simulink model "MECOS_FW_sys"  (R2025b)
settings: Solver=VariableStepAuto  StartTime=0.0  StopTime=1.e-6  RelTol=1e-3
values from neighbouring files (symbols this model uses):
  FPGA_Ts = 1./FPGA_CLK    (= 8e-09)    [choPLL_loop_impl.m]
  FTW_nom_100kHz = round(Fref/FPGA_CLK*2^(Nbit_Cntr+1))    [choPLL_loop_impl.m]
  MECOS_A0 = 1./Bet0    [choPLL_loop_impl.m]
  MECOS_A1 = 2./Bet0    [choPLL_loop_impl.m]
  MECOS_A2 = 1./Bet0    [choPLL_loop_impl.m]
  MECOS_B1 = Bet1/Bet0    [choPLL_loop_impl.m]
  MECOS_B2 = Bet2/Bet0    [choPLL_loop_impl.m]
  MECOS_DF_gain = 0.25* (f_step*Nslits) / (FPGA_CLK/2^(Nbit_Cntr+1))    (= 0.369435906933)    [choPLL_loop_impl.m]
  Nbit_Cntr = 37    [choPLL_loop_impl.m]
libraries: hdlBasic x56, vmcUtilities x1, hdlUtilities x1
settings Model: Creator=valbas  LastModifiedBy=valbas
settings SolverCC: AlgebraicLoopSolver=TrustRegion
settings DebuggingCC: UnconnectedInputMsg=warning  UnconnectedOutputMsg=warning  UnconnectedLineMsg=warning
settings ModelReferenceCC: EnableRefExpFcnMdlSchedulingChecks=on
settings RTWCC: GPUComputeCapability=3.5  DLArmComputeVersion=19.05

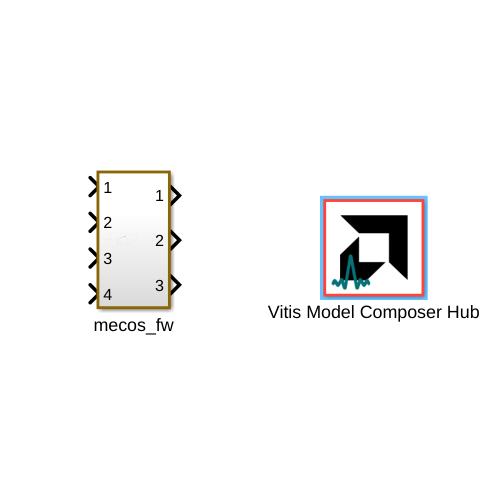
[thumbnail: Simulink's stored preview of the top-level diagram]
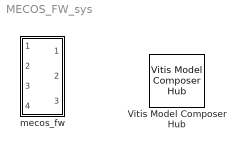
== system MECOS_FW_sys ==
  Vitis Model Composer Hub : vmcUtilities/Vitis Model Composer Hub  Tag=genX  CodeGeneration=off  SubsystemName=mecos_fw  BlockHierPath=MECOS_FW_sys/mecos_fw  CompilationType=HDLCompilation  SubsystemType=HDLNode  ExportTypeV2=IP Catalog  StartColumn=1  NumberOfColumns=1  TargetDirectory=./netlist  exportDesign=on  analyzeDesign=off  validateDesignOnHw=off  ExportType=HDL  IpVendor=xilinx.com  IpLibrary=hls  IpVersion=1.0  IpHWLanguage=Verilog  AieCompilerOptions={}  AieSimulatorOptions={}  CreateTestbench=off  TestbenchStackSize=10  RunRtlSim=off  RunCSim=off  RunAieSim=off  AieSimTimeout=50000  RunAieSimProfiling=off  LaunchVitisAnalyzer=off  PlotOutput=off  RunX86Sim=off  X86SimTimeout=10  GenHwImage=off  GenLibadfXo=on  GenHwValidationCode=off  PlatformType=Not Specified  HwSystemType=Baremetal  HwValidationTarget=hw  ProjDevice=Zynq UltraScale+ ZCU106 Evaluation Platform (xczu7ev-ffvc1156-2-e)  ProjDevicePart=xczu7ev-ffvc1156-2-e  AIEType=None  SamplePeriod=-1  ClockFrequency=200  DataPathParallelism=1  xilinxfamily=zynquplus  part=xczu7ev  speed=-2-e  package=ffvc1156  directory=./code/ip/mecos_fw/src  testbench=off  incr_netlist=off  synthesis_tool=Vivado  clock_wrapper=Clock Enables  dbl_ovrd=According to Block Masks  dcm_input_clock_period=10  sysclk_period=FPGA_Ts*1e9  simulink_period=FPGA_Ts  eval_field=0  IPInfoJsonString="{\"DUTSubsystemName\":\"mecos_fw\",\"HDLSubsystem\":{\"SubsystemName\":\"mecos_fw\",\"IPName\":\"mecos_fw\",\"IPLibrary\":\"ModelComp\",\"IPVendor\":\"MaxIV\",\"IPVersion\":\"1.2\",\"TargetDirectory\":\"./netlist\",\"SubsystemDir\":\"./netlist/ip/mecos_fw\",\"FreqHz\":\"125000000\"},\"SubsystemTag\":\"HDLNode\"}"  LogFileName=/xilinxworks/ZCU106/v2025.2/chopsync/gitcode/modelcomp/netlist/model_composer.log  NThreads=4  IPConfigFile=/tmp/vmctmp-5513881200898270237/MECOS_FW_sys_ipconfig.json
  mecos_fw : Subsystem

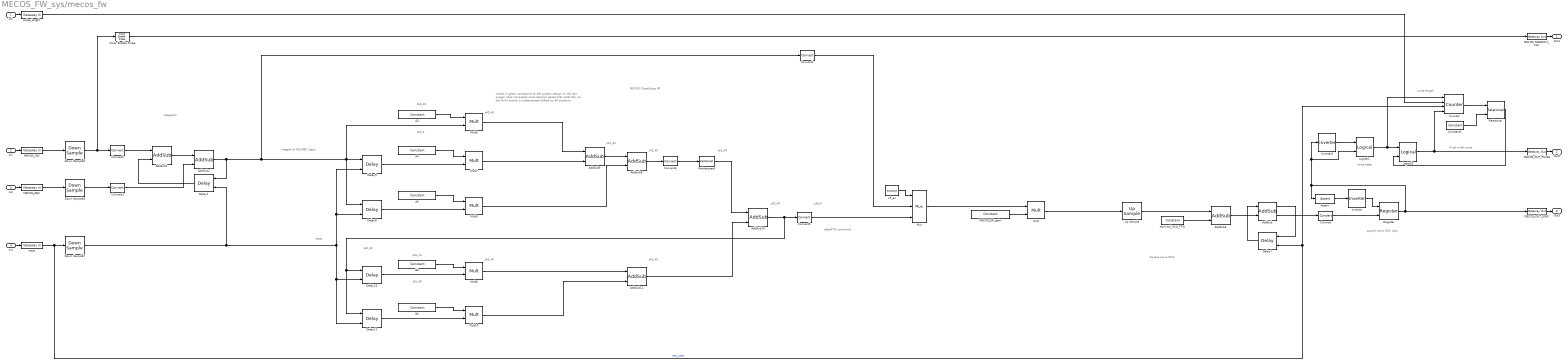
== system MECOS_FW_sys/mecos_fw ==
  note: pulse length
  note: Integrator
  note: Square-wave NCO
  note: s62_40
  note: s26_24
  note: s62_40
  note: s42_40
  note: s40_40
  note: s22_0
  note: s62_40
  note: s62_40
  note: integral of INC/DEC steps
  note: values in green correspond to the system design on the doc;
      | sysgen does not accept more decimal places than total bits,
      | so the AnXn branch is implemented shifted by 40 positions
  note: s18_40
  note: deltaFTW command
  note: MECOS ClosedLoop IIR
  note: s62_40
  note: s62_40
  note: s41_40
  note: reset
  note: s38_0
  note: rising edge
  note: fixed width pulse
  note: square wave 50% duty
  In1 : Inport
  In2 : Inport  Port=2
  In3 : Inport  Port=3
  In4 : Inport  Port=4
  A3 : hdlBasic/Constant  const=MECOS_A0*2^40  gui_display_data_type=Fixed-point  arith_type=Signed (2's comp)  n_bits=18  bin_pt=0  preci_type=Single  exp_width=8  frac_width=24  explicit_period=off  period=1  XmcBlockStatus=1  maskContainerNames=tabcontainer1  block_type=constant  block_config=sysgen:Constant_config
  A4 : hdlBasic/Constant  const=MECOS_A1*2^40  gui_display_data_type=Fixed-point  arith_type=Signed (2's comp)  n_bits=18  bin_pt=0  preci_type=Single  exp_width=8  frac_width=24  explicit_period=off  period=1  XmcBlockStatus=1  maskContainerNames=tabcontainer1  block_type=constant  block_config=sysgen:Constant_config
  A5 : hdlBasic/Constant  const=MECOS_A2*2^40  gui_display_data_type=Fixed-point  arith_type=Signed (2's comp)  n_bits=18  bin_pt=0  preci_type=Single  exp_width=8  frac_width=24  explicit_period=off  period=1  XmcBlockStatus=1  maskContainerNames=tabcontainer1  block_type=constant  block_config=sysgen:Constant_config
  AddSub : hdlBasic/AddSub  mode=Addition  use_carryin=off  use_carryout=on  en=off  latency=0  precision=User Defined  arith_type=Unsigned  n_bits=Nbit_Cntr  bin_pt=0  quantization=Truncate  overflow=Wrap  use_behavioral_HDL=off  hw_selection=Fabric  pipelined=off  XmcBlockStatus=1  maskContainerNames=tabcontainer1  block_type=addsub  block_config=sysgen:Addsub_config
  AddSub1 : hdlBasic/AddSub  mode=Addition  use_carryin=off  use_carryout=off  en=off  latency=0  precision=User Defined  arith_type="Signed  (2's comp)"  n_bits=22  bin_pt=0  quantization="Round  (unbiased: +/- Inf)"  overflow=Saturate  use_behavioral_HDL=off  hw_selection=Fabric  pipelined=off  XmcBlockStatus=1  maskContainerNames=tabcontainer1  block_type=addsub  block_config=sysgen:Addsub_config
  AddSub10 : hdlBasic/AddSub  mode=Subtraction  use_carryin=off  use_carryout=off  en=off  latency=0  precision=User Defined  arith_type="Signed  (2's comp)"  n_bits=62  bin_pt=40  quantization="Round  (unbiased: +/- Inf)"  overflow=Saturate  use_behavioral_HDL=off  hw_selection=Fabric  pipelined=off  XmcBlockStatus=1  maskContainerNames=tabcontainer1  block_type=addsub  block_config=sysgen:Addsub_config
  AddSub11 : hdlBasic/AddSub  mode=Addition  use_carryin=off  use_carryout=off  en=off  latency=0  precision=User Defined  arith_type="Signed  (2's comp)"  n_bits=62  bin_pt=40  quantization="Round  (unbiased: +/- Inf)"  overflow=Saturate  use_behavioral_HDL=off  hw_selection=Fabric  pipelined=off  XmcBlockStatus=1  maskContainerNames=tabcontainer1  block_type=addsub  block_config=sysgen:Addsub_config
  AddSub2 : hdlBasic/AddSub  mode=Subtraction  use_carryin=off  use_carryout=off  en=off  latency=0  precision=User Defined  arith_type="Signed  (2's comp)"  n_bits=22  bin_pt=0  quantization="Round  (unbiased: +/- Inf)"  overflow=Saturate  use_behavioral_HDL=off  hw_selection=Fabric  pipelined=off  XmcBlockStatus=1  maskContainerNames=tabcontainer1  block_type=addsub  block_config=sysgen:Addsub_config
  AddSub3 : hdlBasic/AddSub  mode=Addition  use_carryin=off  use_carryout=off  en=off  latency=1  precision=User Defined  arith_type=Unsigned  n_bits=Nbit_Cntr  bin_pt=0  quantization=Truncate  overflow=Saturate  use_behavioral_HDL=off  hw_selection=Fabric  pipelined=off  XmcBlockStatus=1  maskContainerNames=tabcontainer1  block_type=addsub  block_config=sysgen:Addsub_config
  AddSub8 : hdlBasic/AddSub  mode=Addition  use_carryin=off  use_carryout=off  en=off  latency=0  precision=Full  arith_type=Unsigned  n_bits=16  bin_pt=14  quantization=Truncate  overflow=Wrap  use_behavioral_HDL=off  hw_selection=Fabric  pipelined=off  XmcBlockStatus=1  maskContainerNames=tabcontainer1  block_type=addsub  block_config=sysgen:Addsub_config
  AddSub9 : hdlBasic/AddSub  mode=Addition  use_carryin=off  use_carryout=off  en=off  latency=0  precision=Full  arith_type=Unsigned  n_bits=16  bin_pt=14  quantization=Truncate  overflow=Wrap  use_behavioral_HDL=off  hw_selection=Fabric  pipelined=off  XmcBlockStatus=1  maskContainerNames=tabcontainer1  block_type=addsub  block_config=sysgen:Addsub_config
  Assert : hdlBasic/Assert  assert_type=on  type_source=Explicitly  gui_display_data_type=Boolean  arith_type=Boolean  n_bits=16  bin_pt=14  preci_type=Single  exp_width=8  frac_width=24  assert_rate=off  rate_source=Explicitly  period=1  output_port=on  XmcBlockStatus=1  maskContainerNames=group1  block_type=assert  block_config=sysgen:assert_config  block_width=609  block_height=900
  B3 : hdlBasic/Constant  const=MECOS_B1  gui_display_data_type=Fixed-point  arith_type=Signed (2's comp)  n_bits=26  bin_pt=24  preci_type=Single  exp_width=8  frac_width=24  explicit_period=off  period=1  XmcBlockStatus=1  maskContainerNames=tabcontainer1  block_type=constant  block_config=sysgen:Constant_config
  B4 : hdlBasic/Constant  const=MECOS_B2  gui_display_data_type=Fixed-point  arith_type=Signed (2's comp)  n_bits=26  bin_pt=24  preci_type=Single  exp_width=8  frac_width=24  explicit_period=off  period=1  XmcBlockStatus=1  maskContainerNames=tabcontainer1  block_type=constant  block_config=sysgen:Constant_config
  Clock Enable Probe : hdlUtilities/Clock Enable Probe  inherit_constraints=on  XmcBlockStatus=1  maskContainerNames=group1  block_type=ceprobe  block_config=sysgen:CEProbe_config
  Constant1 : hdlBasic/Constant  const=0  gui_display_data_type=Fixed-point  arith_type=Unsigned  n_bits=10  bin_pt=0  preci_type=Single  exp_width=8  frac_width=24  explicit_period=off  period=1  XmcBlockStatus=1  maskContainerNames=tabcontainer1  block_type=constant  block_config=sysgen:Constant_config
  Convert : hdlBasic/Convert  gui_display_data_type=Boolean  arith_type=Boolean  n_bits=16  bin_pt=14  float_type=Single  exp_bits=8  fraction_bits=24  quantization=Truncate  overflow=Wrap  en=off  latency=1  pipeline=off  XmcBlockStatus=1  maskContainerNames=group2  block_type=convert  block_config=sysgen:Convert_config  block_width=595  block_height=885
  Convert1 : hdlBasic/Convert  gui_display_data_type=Fixed-point  arith_type=Signed (2's comp)  n_bits=38  bin_pt=0  float_type=Single  exp_bits=8  fraction_bits=24  quantization="Round  (unbiased: Even Values)"  overflow=Saturate  en=off  latency=1  pipeline=off  XmcBlockStatus=1  maskContainerNames=group2  block_type=convert  block_config=sysgen:Convert_config  block_width=595  block_height=885
  Convert2 : hdlBasic/Convert  gui_display_data_type=Fixed-point  arith_type=Signed (2's comp)  n_bits=22  bin_pt=0  float_type=Single  exp_bits=8  fraction_bits=24  quantization=Truncate  overflow=Wrap  en=off  latency=0  pipeline=off  XmcBlockStatus=1  maskContainerNames=group2  block_type=convert  block_config=sysgen:Convert_config  block_width=595  block_height=885
  Convert3 : hdlBasic/Convert  gui_display_data_type=Fixed-point  arith_type=Signed (2's comp)  n_bits=22  bin_pt=0  float_type=Single  exp_bits=8  fraction_bits=24  quantization=Truncate  overflow=Wrap  en=off  latency=0  pipeline=off  XmcBlockStatus=1  maskContainerNames=group2  block_type=convert  block_config=sysgen:Convert_config  block_width=595  block_height=885
  Convert5 : hdlBasic/Convert  gui_display_data_type=Fixed-point  arith_type=Signed (2's comp)  n_bits=38  bin_pt=0  float_type=Single  exp_bits=8  fraction_bits=24  quantization="Round  (unbiased: Even Values)"  overflow=Saturate  en=off  latency=1  pipeline=off  XmcBlockStatus=1  maskContainerNames=group2  block_type=convert  block_config=sysgen:Convert_config  block_width=595  block_height=885
  Convert6 : hdlBasic/Convert  gui_display_data_type=Fixed-point  arith_type=Signed (2's comp)  n_bits=62  bin_pt=0  float_type=Single  exp_bits=8  fraction_bits=24  quantization="Round  (unbiased: Even Values)"  overflow=Saturate  en=off  latency=0  pipeline=off  XmcBlockStatus=1  maskContainerNames=group2  block_type=convert  block_config=sysgen:Convert_config  block_width=595  block_height=885
  Counter : hdlBasic/Counter  cnt_type=Free running  cnt_to=Inf  operation=Down  start_count=1  cnt_by_val=1  arith_type=Unsigned  n_bits=10  bin_pt=0  load_pin=on  rst=on  en=on  explicit_period=Explicit  period=FPGA_Ts  use_behavioral_HDL=off  implementation=Fabric  XmcBlockStatus=1  maskContainerNames=group1  block_type=counter  block_config=sysgen:Counter_config  block_width=531  block_height=1023
  Delay{2,7,9..10} (4 alike) : hdlBasic/Delay  rst=on  en=off  latency=1  reg_retiming=off  XmcBlockStatus=1  maskContainerNames=group1  block_type=delay  block_config=sysgen:Delay_config
  Delay11 : hdlBasic/Delay  rst=on  en=off  latency=2  reg_retiming=off  XmcBlockStatus=1  maskContainerNames=group1  block_type=delay  block_config=sysgen:Delay_config
  Delay8 : hdlBasic/Delay  rst=on  en=off  latency=2  reg_retiming=off  XmcBlockStatus=1  maskContainerNames=group1  block_type=delay  block_config=sysgen:Delay_config
  Down Sample5 : hdlBasic/Down Sample  sample_ratio=MECOS_dec  sample_phase="Last Value of Frame  (most efficient)"  en=off  rst=off  latency=1  XmcBlockStatus=1  maskContainerNames=group1  block_type=dsamp  block_config=sysgen:Downsample_config
  Down Sample6 : hdlBasic/Down Sample  sample_ratio=MECOS_dec  sample_phase="Last Value of Frame  (most efficient)"  en=off  rst=off  latency=1  XmcBlockStatus=1  maskContainerNames=group1  block_type=dsamp  block_config=sysgen:Downsample_config
  Down Sample7 : hdlBasic/Down Sample  sample_ratio=MECOS_dec  sample_phase="Last Value of Frame  (most efficient)"  en=off  rst=off  latency=1  XmcBlockStatus=1  maskContainerNames=group1  block_type=dsamp  block_config=sysgen:Downsample_config
  Inverter : hdlBasic/Inverter  en=off  latency=1  XmcBlockStatus=1  maskContainerNames=group2  block_type=inv  block_config=sysgen:Inverter_config
  Inverter3 : hdlBasic/Inverter  en=off  latency=1  XmcBlockStatus=1  maskContainerNames=group2  block_type=inv  block_config=sysgen:Inverter_config
  LP_en : hdlBasic/Constant  const=1  gui_display_data_type=Boolean  arith_type=Boolean  n_bits=18  bin_pt=0  preci_type=Single  exp_width=8  frac_width=24  explicit_period=off  period=1  XmcBlockStatus=1  maskContainerNames=tabcontainer1  block_type=constant  block_config=sysgen:Constant_config
  Logical1 : hdlBasic/Logical  logical_function=AND  inputs=2  en=off  latency=0  precision=Full  arith_type=Unsigned  n_bits=16  bin_pt=0  align_bp=on  overflow=[]  quantization=[]  XmcBlockStatus=1  maskContainerNames=tabcontainer1  block_type=logical  block_config=sysgen:Logical_config
  Logical3 : hdlBasic/Logical  logical_function=OR  inputs=2  en=off  latency=0  precision=Full  arith_type=Unsigned  n_bits=16  bin_pt=0  align_bp=on  overflow=[]  quantization=[]  XmcBlockStatus=1  maskContainerNames=tabcontainer1  block_type=logical  block_config=sysgen:Logical_config
  MECOS_DEC : hdlBasic/Gateway In  gui_display_data_type=Boolean  arith_type=Boolean  n_bits=16  bin_pt=14  preci_type=Single  exp_width=8  frac_width=24  rows=1  columns=1  quantization="Round  (unbiased: +/- Inf)"  overflow=Saturate  period=FPGA_Ts  UseAsADC=off  ADCChannel='1'  interface=None  automatic_assignment=on  address_offset=hex2dec('00')  intf_name=''  intf_description=''  default_value=0  timing_constraint=None  locs_specified=off  LOCs={}  io_standard={}  inherit_from_input=off  hdl_port=on  XmcBlockStatus=1  maskContainerNames=group4  block_type=gatewayin  block_config=sysgen:gateway_in_config  block_width_w=590  block_height_w=620  block_width=640  block_height=850
  MECOS_DF_gain : hdlBasic/Constant  const=MECOS_DF_gain  gui_display_data_type=Fixed-point  arith_type=Signed (2's comp)  n_bits=18  bin_pt=15  preci_type=Single  exp_width=8  frac_width=24  explicit_period=off  period=1  XmcBlockStatus=1  maskContainerNames=tabcontainer1  block_type=constant  block_config=sysgen:Constant_config
  MECOS_INC : hdlBasic/Gateway In  gui_display_data_type=Boolean  arith_type=Boolean  n_bits=16  bin_pt=14  preci_type=Single  exp_width=8  frac_width=24  rows=1  columns=1  quantization="Round  (unbiased: +/- Inf)"  overflow=Saturate  period=FPGA_Ts  UseAsADC=off  ADCChannel='1'  interface=None  automatic_assignment=on  address_offset=hex2dec('00')  intf_name=''  intf_description=''  default_value=0  timing_constraint=None  locs_specified=off  LOCs={}  io_standard={}  inherit_from_input=off  hdl_port=on  XmcBlockStatus=1  maskContainerNames=group4  block_type=gatewayin  block_config=sysgen:gateway_in_config  block_width_w=590  block_height_w=620  block_width=640  block_height=850
  MECOS_OUT_PULSE : hdlBasic/Gateway Out  inherit_from_input=off  bool_to_boolean=off  hdl_port=on  rows=1  columns=1  UseAsDAC=off  DACChannel='1'  interface=None  automatic_assignment=on  address_offset=hex2dec('00')  intf_name=''  intf_description=''  timing_constraint=None  locs_specified=off  LOCs={}  io_standard={}  XmcBlockStatus=1  maskContainerNames=group4  block_type=gatewayout  block_config=sysgen:gateway_out_config  block_width_w=590  block_height_w=620  block_width=620  block_height=750
  MECOS_OUT_SQW : hdlBasic/Gateway Out  inherit_from_input=off  bool_to_boolean=off  hdl_port=on  rows=1  columns=1  UseAsDAC=off  DACChannel='1'  interface=None  automatic_assignment=on  address_offset=hex2dec('00')  intf_name=''  intf_description=''  timing_constraint=None  locs_specified=off  LOCs={}  io_standard={}  XmcBlockStatus=1  maskContainerNames=group4  block_type=gatewayout  block_config=sysgen:gateway_out_config  block_width_w=590  block_height_w=620  block_width=620  block_height=750
  MECOS_READOUT_CLK : hdlBasic/Gateway Out  inherit_from_input=off  bool_to_boolean=off  hdl_port=on  rows=1  columns=1  UseAsDAC=off  DACChannel='1'  interface=None  automatic_assignment=on  address_offset=hex2dec('00')  intf_name=''  intf_description=''  timing_constraint=None  locs_specified=off  LOCs={}  io_standard={}  XmcBlockStatus=1  maskContainerNames=group4  block_type=gatewayout  block_config=sysgen:gateway_out_config  block_width_w=590  block_height_w=620  block_width=620  block_height=750
  Mult : hdlBasic/Mult  precision=User Defined  arith_type="Signed  (2's comp)"  n_bits=38  bin_pt=0  quantization="Round  (unbiased: +/- Inf)"  overflow=Saturate  en=off  latency=0  opt_float=off  fp_mult_usage=No Usage  use_behavioral_HDL=off  opt=Speed  use_embedded=on  optimum_pipeline=off  pipeline=on  use_rpm=on  placement_style=Triangular  XmcBlockStatus=1  maskContainerNames=group1  block_type=mult  block_config=sysgen:Mult_config  block_width=598  block_height=876
  Mult10 : hdlBasic/Mult  precision=User Defined  arith_type="Signed  (2's comp)"  n_bits=62  bin_pt=40  quantization="Round  (unbiased: +/- Inf)"  overflow=Saturate  en=off  latency=0  opt_float=off  fp_mult_usage=No Usage  use_behavioral_HDL=off  opt=Speed  use_embedded=on  optimum_pipeline=off  pipeline=on  use_rpm=on  placement_style=Triangular  XmcBlockStatus=1  maskContainerNames=group1  block_type=mult  block_config=sysgen:Mult_config  block_width=598  block_height=876
  Mult6 : hdlBasic/Mult  precision=Full  arith_type="Signed  (2's comp)"  n_bits=16  bin_pt=14  quantization=Truncate  overflow=Wrap  en=off  latency=0  opt_float=off  fp_mult_usage=No Usage  use_behavioral_HDL=off  opt=Speed  use_embedded=on  optimum_pipeline=off  pipeline=on  use_rpm=on  placement_style=Triangular  XmcBlockStatus=1  maskContainerNames=group1  block_type=mult  block_config=sysgen:Mult_config  block_width=598  block_height=876
  Mult7 : hdlBasic/Mult  precision=Full  arith_type="Signed  (2's comp)"  n_bits=16  bin_pt=14  quantization=Truncate  overflow=Wrap  en=off  latency=0  opt_float=off  fp_mult_usage=No Usage  use_behavioral_HDL=off  opt=Speed  use_embedded=on  optimum_pipeline=off  pipeline=on  use_rpm=on  placement_style=Triangular  XmcBlockStatus=1  maskContainerNames=group1  block_type=mult  block_config=sysgen:Mult_config  block_width=598  block_height=876
  Mult8 : hdlBasic/Mult  precision=User Defined  arith_type="Signed  (2's comp)"  n_bits=62  bin_pt=40  quantization="Round  (unbiased: +/- Inf)"  overflow=Saturate  en=off  latency=0  opt_float=off  fp_mult_usage=No Usage  use_behavioral_HDL=off  opt=Speed  use_embedded=on  optimum_pipeline=off  pipeline=on  use_rpm=on  placement_style=Triangular  XmcBlockStatus=1  maskContainerNames=group1  block_type=mult  block_config=sysgen:Mult_config  block_width=598  block_height=876
  Mult9 : hdlBasic/Mult  precision=Full  arith_type="Signed  (2's comp)"  n_bits=16  bin_pt=14  quantization=Truncate  overflow=Wrap  en=off  latency=0  opt_float=off  fp_mult_usage=No Usage  use_behavioral_HDL=off  opt=Speed  use_embedded=on  optimum_pipeline=off  pipeline=on  use_rpm=on  placement_style=Triangular  XmcBlockStatus=1  maskContainerNames=group1  block_type=mult  block_config=sysgen:Mult_config  block_width=598  block_height=876
  Mux : hdlBasic/Mux  inputs=2  en=off  latency=1  precision=Full  arith_type=Unsigned  n_bits=16  bin_pt=14  quantization=Truncate  overflow=Wrap  XmcBlockStatus=1  maskContainerNames=tabcontainer1  block_type=mux  block_config=sysgen:Mux_config
  Nominal_VCO_FTW : hdlBasic/Constant  const=FTW_nom_100kHz  gui_display_data_type=Fixed-point  arith_type=Signed (2's comp)  n_bits=Nbit_Cntr+1  bin_pt=0  preci_type=Single  exp_width=8  frac_width=24  explicit_period=on  period=FPGA_Ts  XmcBlockStatus=1  maskContainerNames=tabcontainer1  block_type=constant  block_config=sysgen:Constant_config
  Register : hdlBasic/Register  init=0  rst=off  en=on  XmcBlockStatus=1  maskContainerNames=tabcontainer1  block_type=register  block_config=sysgen:Register_config
  Reinterpret4 : hdlBasic/Reinterpret  force_arith_type=off  arith_type=Unsigned  force_bin_pt=on  bin_pt=40  XmcBlockStatus=1  maskContainerNames=group1  block_type=reinterpret  block_config=sysgen:Reinterpret_config
  Relational : hdlBasic/Relational  mode=a!=b  op_type=Bool  en=off  latency=0  XmcBlockStatus=1  maskContainerNames=tabcontainer1  block_type=relational  block_config=sysgen:Relational_config
  Up Sample : hdlBasic/Up Sample  sample_ratio=MECOS_dec  copy_samples=on  en=off  latency=1  XmcBlockStatus=1  maskContainerNames=group1  block_type=usamp  block_config=sysgen:Upsample_config
  pulse_length : hdlBasic/Gateway In  gui_display_data_type=Fixed-point  arith_type=Unsigned  n_bits=10  bin_pt=0  preci_type=Single  exp_width=8  frac_width=24  rows=1  columns=1  quantization="Round  (unbiased: +/- Inf)"  overflow=Saturate  period=FPGA_Ts  UseAsADC=off  ADCChannel='1'  interface=None  automatic_assignment=on  address_offset=hex2dec('00')  intf_name=''  intf_description=''  default_value=0  timing_constraint=None  locs_specified=off  LOCs={}  io_standard={}  inherit_from_input=off  hdl_port=on  XmcBlockStatus=1  maskContainerNames=group4  block_type=gatewayin  block_config=sysgen:gateway_in_config  block_width_w=590  block_height_w=620  block_width=640  block_height=850
  reset : hdlBasic/Gateway In  gui_display_data_type=Boolean  arith_type=Boolean  n_bits=16  bin_pt=14  preci_type=Single  exp_width=8  frac_width=24  rows=1  columns=1  quantization="Round  (unbiased: +/- Inf)"  overflow=Saturate  period=FPGA_Ts  UseAsADC=off  ADCChannel='1'  interface=None  automatic_assignment=on  address_offset=hex2dec('00')  intf_name=''  intf_description=''  default_value=0  timing_constraint=None  locs_specified=off  LOCs={}  io_standard={}  inherit_from_input=off  hdl_port=on  XmcBlockStatus=1  maskContainerNames=group4  block_type=gatewayin  block_config=sysgen:gateway_in_config  block_width_w=590  block_height_w=620  block_width=640  block_height=850
  Out1 : Outport
  Out2 : Outport  Port=2
  Out3 : Outport  Port=3
  wires:
  In1/1 -> pulse_length/1
  Mux/1 -> Mult/1
  B3/1 -> Mult8/1
  Clock Enable Probe/1 -> MECOS_READOUT_CLK/1
  Mult10/1 -> AddSub11/2
  Up Sample/1 -> AddSub3/1
  Delay8/1 -> Mult9/2
  AddSub11/1 -> AddSub10/2
  Delay7/1 -> AddSub/1
  Logical3/1 -> MECOS_OUT_PULSE/1, Counter/4
  Delay11/1 -> Mult10/2
  MECOS_DF_gain/1 -> Mult/2
  A3/1 -> Mult6/1
  Reinterpret4/1 -> AddSub10/1
  Delay2/1 -> AddSub1/2
  B4/1 -> Mult10/1
  A4/1 -> Mult7/1
  Mult6/1 -> AddSub9/1
  MECOS_OUT_SQW/1 -> Out3/1
  AddSub10/1 -> Delay10/1, Delay11/1, Convert5/1
  AddSub/2 -> Convert/1
  Assert/1 -> Inverter/1
  Down Sample6/1 -> Convert3/1
  AddSub/1 -> Delay7/1
  AddSub3/1 -> AddSub/2
  Down Sample5/1 -> Clock Enable Probe/1, Convert2/1
  Inverter/1 -> Register/1
  Convert1/1 -> Mux/2
  AddSub9/1 -> AddSub8/1
  reset/1 -> Delay7/2, Counter/3, Down Sample7/1  "RES_125M"
  pulse_length/1 -> Counter/2
  Constant1/1 -> Relational/2
  Mult/1 -> Up Sample/1
  In2/1 -> MECOS_INC/1
  Delay9/1 -> Mult7/2
  Counter/1 -> Relational/1
  Mult8/1 -> AddSub11/1
  MECOS_OUT_PULSE/1 -> Out2/1
  Nominal_VCO_FTW/1 -> AddSub3/2
  Logical1/1 -> Logical3/1, Counter/1
  In3/1 -> MECOS_DEC/1
  Convert2/1 -> AddSub1/1
  MECOS_INC/1 -> Down Sample5/1
  Relational/1 -> Logical3/2
  Convert/1 -> Register/2
  MECOS_DEC/1 -> Down Sample6/1
  A5/1 -> Mult9/1
  Delay10/1 -> Mult8/2
  LP_en/1 -> Mux/1
  Down Sample7/1 -> Delay11/2, Delay10/2, Delay9/2, Delay8/2, Delay2/2
  AddSub8/1 -> Convert6/1
  AddSub1/1 -> AddSub2/1
  Convert6/1 -> Reinterpret4/1
  Mult9/1 -> AddSub8/2
  MECOS_READOUT_CLK/1 -> Out1/1
  Register/1 -> Assert/1, Logical1/2, Inverter3/1, MECOS_OUT_SQW/1
  Inverter3/1 -> Logical1/1
  Mult7/1 -> AddSub9/2
  Convert3/1 -> AddSub2/2
  In4/1 -> reset/1
  AddSub2/1 -> Delay2/1, Delay8/1, Mult6/2, Delay9/1, Convert1/1
  Convert5/1 -> Mux/3
